simulink model "ElectricalSystem_Test"  (R2019b)
settings: Solver=VariableStepAuto  StartTime=0.0  StopTime=inf  RelTol=1e-3
PostLoadFcn:
  | set_up_test_model
undefined symbols (not defined in the file): AC1CB, AC2CB, AirSupplyIC, APSCB, ATCCabActivation, ATCZeroSpeed, ATOTBDemand, Audio, BLCB, Braking, CECB, CELCB, Class, CMCCB, CRSBCB, CSACB, CSBCB, CSCCB, DeadmanSafetyDevice, DIOCB1, DIOCB2, DLCB, DMICB, Doors, DPLCB, DRCB, EIVIB, ElectricalSystemInput, ElectricalTrainConnection, ElectricalUnitConnection, EmergencyBrakePB, Enabled, ForwardDirection, GrossMass, HasCab, HasMainCompressor, HasMotor, HasPanto, HeadlightSwitch, Height, HLCB, HornPB, ILCB1, ILCB2, IsDM1, IsDM2, IsM1, IsM2, IsT1, IsT2, LeftSideDoorOpen, Length, LoadingMass, MainReservoirPressureSwitch, MasterKeySwitch, MaxVehicles, ModeSelector, NotImmobilise, NotSafetyBrake, NVICB ... (+47)
libraries: TestBenchLib x81
(part 2 of 2)

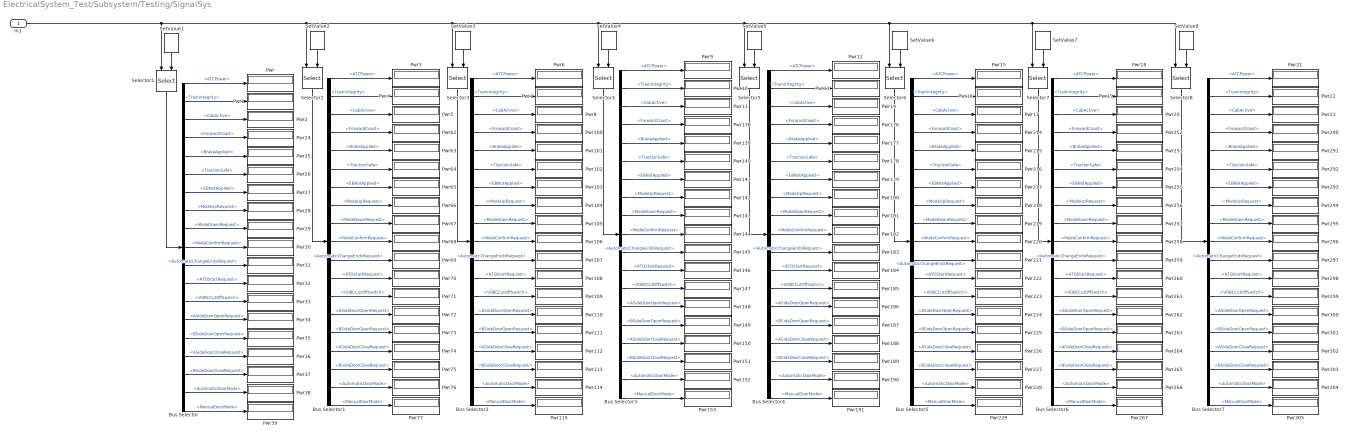
== system ElectricalSystem_Test/Subsystem/Testing/SignalSys ==
  In1 : Inport
  Bus Selector{,1..7} (8 alike) : BusSelector  OutputSignals=SignalSys.ATCPower,SignalSys.TrainIntegrity,SignalSys.CabActive,SignalSys.ForwardCoast,SignalSys.BrakeApplied,SignalSys.TractionSafe,SignalSys.EBNotApplied,SignalSys.ModeUpRequest,SignalSys.ModeDownRequest,SignalSys.ModeConfirmRequest,SignalSys.AutomaticChangeEndsRequest,SignalSys.ATOStartRequest,SignalSys.VOBCCutOffSwitch,SignalSys.ASideDoorOpenRequest,SignalSys.BSideDoorOpenRequest,SignalSys.ASideDoorCloseRequest,SignalSys.BSideDoorCloseRequest,SignalSys.AutomaticDoorMode,SignalSys.ManualDoorMode
  Pwr{,1..39,62..77,100..115,138..153,176..191,214..229,252..267,290..305} (152 alike) : Display
  Selector{1..8} (8 alike) : Selector  InputPortWidth=8  IndexOptions=Index vector (port)  Indices=[1 3]  OutputSizes=1
  SetValue1 : TestBenchLib/SetValue  value=1  init_value=1  WorkspaceVarName=0
      settings: SourceProductName=Sydac Utilities
  SetValue2 : TestBenchLib/SetValue  value=2  init_value=2  WorkspaceVarName=0
      settings: SourceProductName=Sydac Utilities
  SetValue3 : TestBenchLib/SetValue  value=3  init_value=3  WorkspaceVarName=0
      settings: SourceProductName=Sydac Utilities
  SetValue4 : TestBenchLib/SetValue  value=4  init_value=4  WorkspaceVarName=0
      settings: SourceProductName=Sydac Utilities
  SetValue5 : TestBenchLib/SetValue  value=5  init_value=5  WorkspaceVarName=0
      settings: SourceProductName=Sydac Utilities
  SetValue6 : TestBenchLib/SetValue  value=6  init_value=6  WorkspaceVarName=0
      settings: SourceProductName=Sydac Utilities
  SetValue7 : TestBenchLib/SetValue  value=7  init_value=7  WorkspaceVarName=0
      settings: SourceProductName=Sydac Utilities
  SetValue8 : TestBenchLib/SetValue  value=8  init_value=8  WorkspaceVarName=0
      settings: SourceProductName=Sydac Utilities
  wires:
  Selector1/1 -> Bus Selector/1
  SetValue1/1 -> Selector1/2
  Bus Selector/1 -> Pwr/1  "<ATCPower>"
  Bus Selector/2 -> Pwr1/1  "<TrainIntegrity>"
  Bus Selector/3 -> Pwr2/1  "<CabActive>"
  SetValue2/1 -> Selector2/2
  SetValue3/1 -> Selector3/2
  SetValue4/1 -> Selector4/2
  SetValue5/1 -> Selector5/2
  In1/1 -> Selector8/1, Selector7/1, Selector6/1, Selector5/1, Selector4/1, Selector3/1, Selector2/1, Selector1/1
  SetValue6/1 -> Selector6/2
  SetValue7/1 -> Selector7/2
  SetValue8/1 -> Selector8/2
  Bus Selector/4 -> Pwr24/1  "<ForwardCoast>"
  Bus Selector/5 -> Pwr25/1  "<BrakeApplied>"
  Bus Selector/6 -> Pwr26/1  "<TractionSafe>"
  Bus Selector/7 -> Pwr27/1  "<EBNotApplied>"
  Bus Selector/8 -> Pwr28/1  "<ModeUpRequest>"
  Bus Selector/9 -> Pwr29/1  "<ModeDownRequest>"
  Bus Selector/10 -> Pwr30/1  "<ModeConfirmRequest>"
  Bus Selector/11 -> Pwr31/1  "<AutomaticChangeEndsRequest>"
  Bus Selector/12 -> Pwr32/1  "<ATOStartRequest>"
  Bus Selector/13 -> Pwr33/1  "<VOBCCutOffSwitch>"
  Bus Selector/14 -> Pwr34/1  "<ASideDoorOpenRequest>"
  Bus Selector/15 -> Pwr35/1  "<BSideDoorOpenRequest>"
  Bus Selector/16 -> Pwr36/1  "<ASideDoorCloseRequest>"
  Bus Selector/17 -> Pwr37/1  "<BSideDoorCloseRequest>"
  Bus Selector/18 -> Pwr38/1  "<AutomaticDoorMode>"
  Bus Selector/19 -> Pwr39/1  "<ManualDoorMode>"
  Bus Selector1/4 -> Pwr62/1  "<ForwardCoast>"
  Bus Selector1/19 -> Pwr77/1  "<ManualDoorMode>"
  Bus Selector1/17 -> Pwr75/1  "<BSideDoorCloseRequest>"
  Bus Selector1/18 -> Pwr76/1  "<AutomaticDoorMode>"
  Bus Selector1/14 -> Pwr72/1  "<ASideDoorOpenRequest>"
  Bus Selector1/16 -> Pwr74/1  "<ASideDoorCloseRequest>"
  Bus Selector1/15 -> Pwr73/1  "<BSideDoorOpenRequest>"
  Bus Selector1/11 -> Pwr69/1  "<AutomaticChangeEndsRequest>"
  Bus Selector1/13 -> Pwr71/1  "<VOBCCutOffSwitch>"
  Bus Selector1/12 -> Pwr70/1  "<ATOStartRequest>"
  Bus Selector1/9 -> Pwr67/1  "<ModeDownRequest>"
  Bus Selector1/8 -> Pwr66/1  "<ModeUpRequest>"
  Bus Selector1/7 -> Pwr65/1  "<EBNotApplied>"
  Bus Selector1/6 -> Pwr64/1  "<TractionSafe>"
  Bus Selector1/2 -> Pwr4/1  "<TrainIntegrity>"
  Bus Selector1/10 -> Pwr68/1  "<ModeConfirmRequest>"
  Bus Selector1/3 -> Pwr5/1  "<CabActive>"
  Bus Selector1/1 -> Pwr3/1  "<ATCPower>"
  Bus Selector1/5 -> Pwr63/1  "<BrakeApplied>"
  Selector2/1 -> Bus Selector1/1
  Bus Selector2/4 -> Pwr100/1  "<ForwardCoast>"
  Bus Selector2/19 -> Pwr115/1  "<ManualDoorMode>"
  Bus Selector2/17 -> Pwr113/1  "<BSideDoorCloseRequest>"
  Bus Selector2/18 -> Pwr114/1  "<AutomaticDoorMode>"
  Bus Selector2/14 -> Pwr110/1  "<ASideDoorOpenRequest>"
  Bus Selector2/16 -> Pwr112/1  "<ASideDoorCloseRequest>"
  Bus Selector2/15 -> Pwr111/1  "<BSideDoorOpenRequest>"
  Bus Selector2/11 -> Pwr107/1  "<AutomaticChangeEndsRequest>"
  Bus Selector2/13 -> Pwr109/1  "<VOBCCutOffSwitch>"
  Bus Selector2/12 -> Pwr108/1  "<ATOStartRequest>"
  Bus Selector2/9 -> Pwr105/1  "<ModeDownRequest>"
  Bus Selector2/8 -> Pwr104/1  "<ModeUpRequest>"
  Bus Selector2/7 -> Pwr103/1  "<EBNotApplied>"
  Bus Selector2/6 -> Pwr102/1  "<TractionSafe>"
  Bus Selector2/2 -> Pwr7/1  "<TrainIntegrity>"
  Bus Selector2/10 -> Pwr106/1  "<ModeConfirmRequest>"
  Bus Selector2/3 -> Pwr8/1  "<CabActive>"
  Bus Selector2/1 -> Pwr6/1  "<ATCPower>"
  Bus Selector2/5 -> Pwr101/1  "<BrakeApplied>"
  Selector3/1 -> Bus Selector2/1
  Bus Selector3/4 -> Pwr138/1  "<ForwardCoast>"
  Bus Selector3/19 -> Pwr153/1  "<ManualDoorMode>"
  Bus Selector3/17 -> Pwr151/1  "<BSideDoorCloseRequest>"
  Bus Selector3/18 -> Pwr152/1  "<AutomaticDoorMode>"
  Bus Selector3/14 -> Pwr148/1  "<ASideDoorOpenRequest>"
  Bus Selector3/16 -> Pwr150/1  "<ASideDoorCloseRequest>"
  Bus Selector3/15 -> Pwr149/1  "<BSideDoorOpenRequest>"
  Bus Selector3/11 -> Pwr145/1  "<AutomaticChangeEndsRequest>"
  Bus Selector3/13 -> Pwr147/1  "<VOBCCutOffSwitch>"
  Bus Selector3/12 -> Pwr146/1  "<ATOStartRequest>"
  Bus Selector3/9 -> Pwr143/1  "<ModeDownRequest>"
  Bus Selector3/8 -> Pwr142/1  "<ModeUpRequest>"
  Bus Selector3/7 -> Pwr141/1  "<EBNotApplied>"
  Bus Selector3/6 -> Pwr140/1  "<TractionSafe>"
  Bus Selector3/2 -> Pwr10/1  "<TrainIntegrity>"
  Bus Selector3/10 -> Pwr144/1  "<ModeConfirmRequest>"
  Bus Selector3/3 -> Pwr11/1  "<CabActive>"
  Bus Selector3/1 -> Pwr9/1  "<ATCPower>"
  Bus Selector3/5 -> Pwr139/1  "<BrakeApplied>"
  Selector4/1 -> Bus Selector3/1
  Bus Selector4/4 -> Pwr176/1  "<ForwardCoast>"
  Bus Selector4/19 -> Pwr191/1  "<ManualDoorMode>"
  Bus Selector4/17 -> Pwr189/1  "<BSideDoorCloseRequest>"
  Bus Selector4/18 -> Pwr190/1  "<AutomaticDoorMode>"
  Bus Selector4/14 -> Pwr186/1  "<ASideDoorOpenRequest>"
  Bus Selector4/16 -> Pwr188/1  "<ASideDoorCloseRequest>"
  Bus Selector4/15 -> Pwr187/1  "<BSideDoorOpenRequest>"
  Bus Selector4/11 -> Pwr183/1  "<AutomaticChangeEndsRequest>"
  Bus Selector4/13 -> Pwr185/1  "<VOBCCutOffSwitch>"
  Bus Selector4/12 -> Pwr184/1  "<ATOStartRequest>"
  Bus Selector4/9 -> Pwr181/1  "<ModeDownRequest>"
  Bus Selector4/8 -> Pwr180/1  "<ModeUpRequest>"
  Bus Selector4/7 -> Pwr179/1  "<EBNotApplied>"
  Bus Selector4/6 -> Pwr178/1  "<TractionSafe>"
  Bus Selector4/2 -> Pwr13/1  "<TrainIntegrity>"
  Bus Selector4/10 -> Pwr182/1  "<ModeConfirmRequest>"
  Bus Selector4/3 -> Pwr14/1  "<CabActive>"
  Bus Selector4/1 -> Pwr12/1  "<ATCPower>"
  Bus Selector4/5 -> Pwr177/1  "<BrakeApplied>"
  Bus Selector5/4 -> Pwr214/1  "<ForwardCoast>"
  Bus Selector5/19 -> Pwr229/1  "<ManualDoorMode>"
  Bus Selector5/17 -> Pwr227/1  "<BSideDoorCloseRequest>"
  Bus Selector5/18 -> Pwr228/1  "<AutomaticDoorMode>"
  Bus Selector5/14 -> Pwr224/1  "<ASideDoorOpenRequest>"
  Bus Selector5/16 -> Pwr226/1  "<ASideDoorCloseRequest>"
  Bus Selector5/15 -> Pwr225/1  "<BSideDoorOpenRequest>"
  Bus Selector5/11 -> Pwr221/1  "<AutomaticChangeEndsRequest>"
  Bus Selector5/13 -> Pwr223/1  "<VOBCCutOffSwitch>"
  Bus Selector5/12 -> Pwr222/1  "<ATOStartRequest>"
  Bus Selector5/9 -> Pwr219/1  "<ModeDownRequest>"
  Bus Selector5/8 -> Pwr218/1  "<ModeUpRequest>"
  Bus Selector5/7 -> Pwr217/1  "<EBNotApplied>"
  Bus Selector5/6 -> Pwr216/1  "<TractionSafe>"
  Bus Selector5/2 -> Pwr16/1  "<TrainIntegrity>"
  Bus Selector5/10 -> Pwr220/1  "<ModeConfirmRequest>"
  Bus Selector5/3 -> Pwr17/1  "<CabActive>"
  Bus Selector5/1 -> Pwr15/1  "<ATCPower>"
  Bus Selector5/5 -> Pwr215/1  "<BrakeApplied>"
  Selector6/1 -> Bus Selector5/1
  Bus Selector6/4 -> Pwr252/1  "<ForwardCoast>"
  Bus Selector6/19 -> Pwr267/1  "<ManualDoorMode>"
  Bus Selector6/17 -> Pwr265/1  "<BSideDoorCloseRequest>"
  Bus Selector6/18 -> Pwr266/1  "<AutomaticDoorMode>"
  Bus Selector6/14 -> Pwr262/1  "<ASideDoorOpenRequest>"
  Bus Selector6/16 -> Pwr264/1  "<ASideDoorCloseRequest>"
  Bus Selector6/15 -> Pwr263/1  "<BSideDoorOpenRequest>"
  Bus Selector6/11 -> Pwr259/1  "<AutomaticChangeEndsRequest>"
  Bus Selector6/13 -> Pwr261/1  "<VOBCCutOffSwitch>"
  Bus Selector6/12 -> Pwr260/1  "<ATOStartRequest>"
  Bus Selector6/9 -> Pwr257/1  "<ModeDownRequest>"
  Bus Selector6/8 -> Pwr256/1  "<ModeUpRequest>"
  Bus Selector6/7 -> Pwr255/1  "<EBNotApplied>"
  Bus Selector6/6 -> Pwr254/1  "<TractionSafe>"
  Bus Selector6/2 -> Pwr19/1  "<TrainIntegrity>"
  Bus Selector6/10 -> Pwr258/1  "<ModeConfirmRequest>"
  Bus Selector6/3 -> Pwr20/1  "<CabActive>"
  Bus Selector6/1 -> Pwr18/1  "<ATCPower>"
  Bus Selector6/5 -> Pwr253/1  "<BrakeApplied>"
  Selector7/1 -> Bus Selector6/1
  Bus Selector7/4 -> Pwr290/1  "<ForwardCoast>"
  Bus Selector7/19 -> Pwr305/1  "<ManualDoorMode>"
  Bus Selector7/17 -> Pwr303/1  "<BSideDoorCloseRequest>"
  Bus Selector7/18 -> Pwr304/1  "<AutomaticDoorMode>"
  Bus Selector7/14 -> Pwr300/1  "<ASideDoorOpenRequest>"
  Bus Selector7/16 -> Pwr302/1  "<ASideDoorCloseRequest>"
  Bus Selector7/15 -> Pwr301/1  "<BSideDoorOpenRequest>"
  Bus Selector7/11 -> Pwr297/1  "<AutomaticChangeEndsRequest>"
  Bus Selector7/13 -> Pwr299/1  "<VOBCCutOffSwitch>"
  Bus Selector7/12 -> Pwr298/1  "<ATOStartRequest>"
  Bus Selector7/9 -> Pwr295/1  "<ModeDownRequest>"
  Bus Selector7/8 -> Pwr294/1  "<ModeUpRequest>"
  Bus Selector7/7 -> Pwr293/1  "<EBNotApplied>"
  Bus Selector7/6 -> Pwr292/1  "<TractionSafe>"
  Bus Selector7/2 -> Pwr22/1  "<TrainIntegrity>"
  Bus Selector7/10 -> Pwr296/1  "<ModeConfirmRequest>"
  Bus Selector7/3 -> Pwr23/1  "<CabActive>"
  Bus Selector7/1 -> Pwr21/1  "<ATCPower>"
  Bus Selector7/5 -> Pwr291/1  "<BrakeApplied>"
  Selector8/1 -> Bus Selector7/1
  Selector5/1 -> Bus Selector4/1

== system ElectricalSystem_Test/Subsystem/Testing/Subsystem ==
  In1 : Inport
  Bus Creator : BusCreator  Inputs=OutputControlStates,Traction,Braking,TCMS,Pneumatics,SignalSys,Doors,Audio
  For Each Subsystem : Subsystem  TreatAsAtomicUnit=on
  Out1 : Outport
  wires:
  In1/1 -> For Each Subsystem/1(In1)
  For Each Subsystem/1(Out1) -> Bus Creator/1  "OutputControlStates"
  For Each Subsystem/2(Out2) -> Bus Creator/2  "Traction"
  For Each Subsystem/3(Out3) -> Bus Creator/3  "Braking"
  For Each Subsystem/4(Out5) -> Bus Creator/4  "TCMS"
  For Each Subsystem/5(Out6) -> Bus Creator/5  "Pneumatics"
  For Each Subsystem/6(Out7) -> Bus Creator/6  "SignalSys"
  For Each Subsystem/7(Out8) -> Bus Creator/7  "Doors"
  Bus Creator/1 -> Out1/1
  For Each Subsystem/8(Out4) -> Bus Creator/8  "Audio"

== system ElectricalSystem_Test/Subsystem/Testing/Subsystem1 ==
  In1 : Inport  Partition=on  PartitionDimension=1  PartitionWidth=1  PartitionOffset=0
  In2 : Inport  Port=2  Partition=on  PartitionDimension=1  PartitionWidth=1  PartitionOffset=0
  Bus Assignment4 : BusAssignment  AssignedSignals=ElectricalUnitConnection,ElectricalTrainConnection
  Constant5 : Constant  Value=0  OutDataTypeStr=Bus: BD_ElectricalSystem_In_Vehicle_Coupling
  For Each : ForEach  DisableCoverage=on
  Out1 : Outport  ConcatenationDimension=1
  wires:
  Constant5/1 -> Bus Assignment4/1
  In1/1 -> Bus Assignment4/2
  Bus Assignment4/1 -> Out1/1
  In2/1 -> Bus Assignment4/3

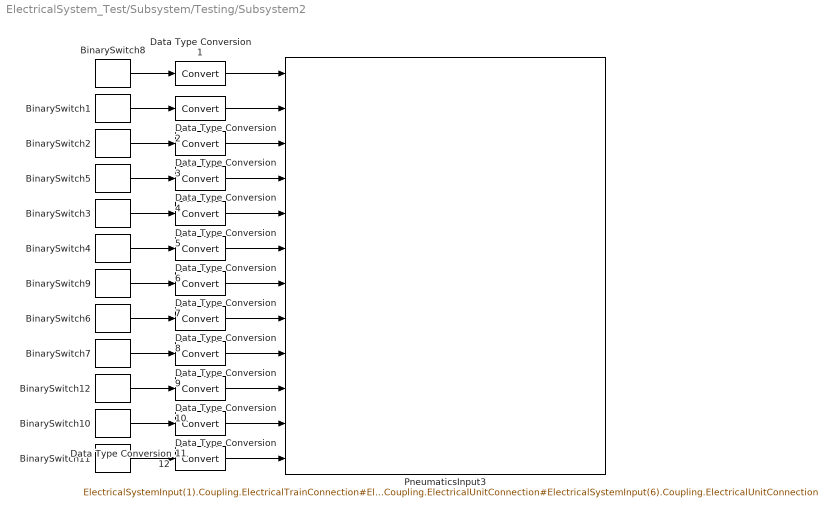
== system ElectricalSystem_Test/Subsystem/Testing/Subsystem2 ==
  BinarySwitch{1..7,10..11} (9 alike) : TestBenchLib/BinarySwitch  value=1  init_value=1  block_colour=[0 1 0]  WorkspaceVarName=0
      settings: SourceProductName=Sydac Utilities
  BinarySwitch12 : TestBenchLib/BinarySwitch  value=0  init_value=0  block_colour=[0 1 0]  WorkspaceVarName=0
      settings: SourceProductName=Sydac Utilities
  BinarySwitch8 : TestBenchLib/BinarySwitch  value=0  init_value=0  block_colour=[0 1 0]  WorkspaceVarName=0
      settings: SourceProductName=Sydac Utilities
  BinarySwitch9 : TestBenchLib/BinarySwitch  value=0  init_value=0  block_colour=[0 1 0]  WorkspaceVarName=0
      settings: SourceProductName=Sydac Utilities
  Data Type Conversion{1..12} (12 alike) : DataTypeConversion
  PneumaticsInput3 : DataStoreWrite  DataStoreName=ElectricalSystemInput  DataStoreElements=ElectricalSystemInput(1).Coupling.ElectricalTrainConnection#ElectricalSystemInput(2).Coupling.ElectricalTrainConnection#ElectricalSystemInput(3).Coupling.ElectricalTrainConnection#ElectricalSystemInput(4).Coupling.ElectricalTrainConnection#ElectricalSystemInput(5).Coupling.ElectricalTrainConnection#ElectricalSystemInput(6).Coupling.ElectricalTrainConnection#ElectricalSystemInput(1).Coupling.ElectricalUnitConnection#ElectricalSystemInput(2).Coupling.ElectricalUnitConnection#ElectricalSystemInput(3).Coupling.ElectricalUnitConnection#ElectricalSystemInput(4).Coupling.ElectricalUnitConnection#ElectricalSystemInput(5).Coupling.ElectricalUnitConnection#ElectricalSystemInput(6).Coupling.ElectricalUnitConnection
  wires:
  Data Type Conversion1/1 -> PneumaticsInput3/1
  BinarySwitch8/1 -> Data Type Conversion1/1
  BinarySwitch1/1 -> Data Type Conversion2/1
  Data Type Conversion2/1 -> PneumaticsInput3/2
  BinarySwitch2/1 -> Data Type Conversion3/1
  Data Type Conversion3/1 -> PneumaticsInput3/3
  Data Type Conversion6/1 -> PneumaticsInput3/6
  BinarySwitch4/1 -> Data Type Conversion6/1
  Data Type Conversion5/1 -> PneumaticsInput3/5
  BinarySwitch3/1 -> Data Type Conversion5/1
  BinarySwitch5/1 -> Data Type Conversion4/1
  Data Type Conversion4/1 -> PneumaticsInput3/4
  BinarySwitch9/1 -> Data Type Conversion7/1
  BinarySwitch6/1 -> Data Type Conversion8/1
  BinarySwitch7/1 -> Data Type Conversion9/1
  Data Type Conversion9/1 -> PneumaticsInput3/9
  Data Type Conversion8/1 -> PneumaticsInput3/8
  Data Type Conversion7/1 -> PneumaticsInput3/7
  Data Type Conversion11/1 -> PneumaticsInput3/11
  Data Type Conversion12/1 -> PneumaticsInput3/12
  BinarySwitch11/1 -> Data Type Conversion12/1
  BinarySwitch10/1 -> Data Type Conversion11/1
  Data Type Conversion10/1 -> PneumaticsInput3/10
  BinarySwitch12/1 -> Data Type Conversion10/1

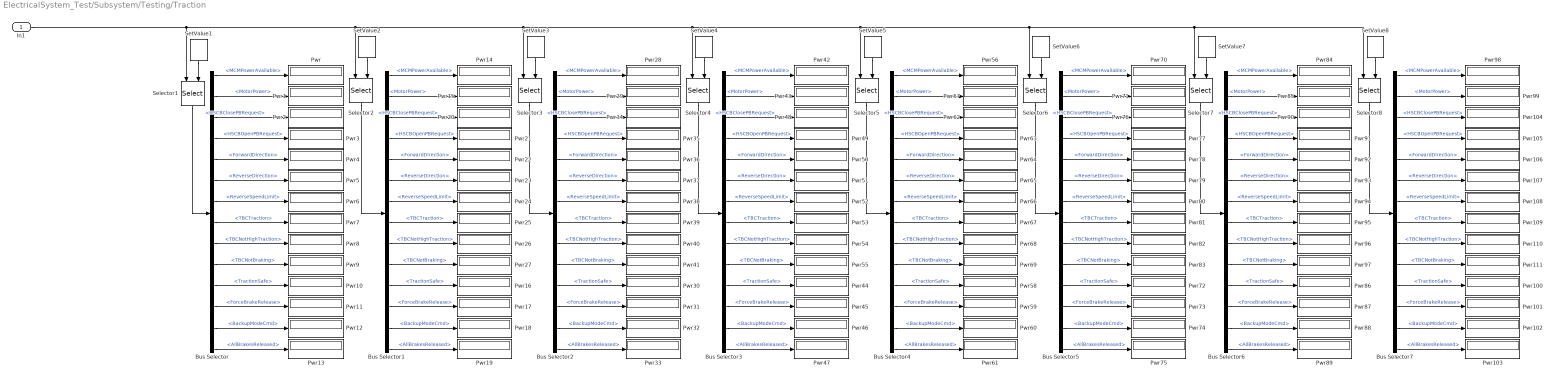
== system ElectricalSystem_Test/Subsystem/Testing/Traction ==
  In1 : Inport
  Bus Selector{,1..7} (8 alike) : BusSelector  OutputSignals=Traction.MCMPowerAvailable,Traction.MotorPower,Traction.HSCBClosePBRequest,Traction.HSCBOpenPBRequest,Traction.ForwardDirection,Traction.ReverseDirection,Traction.ReverseSpeedLimit,Traction.TBCTraction,Traction.TBCNotHighTraction,Traction.TBCNotBraking,Traction.TractionSafe,Traction.ForceBrakeRelease,Traction.BackupModeCmd,Traction.AllBrakesReleased
  Pwr{,1..111} (112 alike) : Display
  Selector{1..8} (8 alike) : Selector  InputPortWidth=8  IndexOptions=Index vector (port)  Indices=[1 3]  OutputSizes=1
  SetValue1 : TestBenchLib/SetValue  value=1  init_value=1  WorkspaceVarName=0
      settings: SourceProductName=Sydac Utilities
  SetValue2 : TestBenchLib/SetValue  value=2  init_value=2  WorkspaceVarName=0
      settings: SourceProductName=Sydac Utilities
  SetValue3 : TestBenchLib/SetValue  value=3  init_value=3  WorkspaceVarName=0
      settings: SourceProductName=Sydac Utilities
  SetValue4 : TestBenchLib/SetValue  value=4  init_value=4  WorkspaceVarName=0
      settings: SourceProductName=Sydac Utilities
  SetValue5 : TestBenchLib/SetValue  value=5  init_value=5  WorkspaceVarName=0
      settings: SourceProductName=Sydac Utilities
  SetValue6 : TestBenchLib/SetValue  value=6  init_value=6  WorkspaceVarName=0
      settings: SourceProductName=Sydac Utilities
  SetValue7 : TestBenchLib/SetValue  value=7  init_value=7  WorkspaceVarName=0
      settings: SourceProductName=Sydac Utilities
  SetValue8 : TestBenchLib/SetValue  value=8  init_value=8  WorkspaceVarName=0
      settings: SourceProductName=Sydac Utilities
  wires:
  Selector1/1 -> Bus Selector/1
  SetValue1/1 -> Selector1/2
  Bus Selector/1 -> Pwr/1  "<MCMPowerAvailable>"
  Bus Selector/2 -> Pwr1/1  "<MotorPower>"
  Bus Selector/3 -> Pwr2/1  "<HSCBClosePBRequest>"
  Bus Selector/4 -> Pwr3/1  "<HSCBOpenPBRequest>"
  Bus Selector/5 -> Pwr4/1  "<ForwardDirection>"
  Bus Selector/6 -> Pwr5/1  "<ReverseDirection>"
  Bus Selector/7 -> Pwr6/1  "<ReverseSpeedLimit>"
  Bus Selector/8 -> Pwr7/1  "<TBCTraction>"
  Bus Selector/9 -> Pwr8/1  "<TBCNotHighTraction>"
  Bus Selector/10 -> Pwr9/1  "<TBCNotBraking>"
  Bus Selector/11 -> Pwr10/1  "<TractionSafe>"
  Bus Selector/12 -> Pwr11/1  "<ForceBrakeRelease>"
  Bus Selector/13 -> Pwr12/1  "<BackupModeCmd>"
  Bus Selector/14 -> Pwr13/1  "<AllBrakesReleased>"
  Bus Selector1/14 -> Pwr19/1  "<AllBrakesReleased>"
  Bus Selector1/13 -> Pwr18/1  "<BackupModeCmd>"
  Bus Selector1/12 -> Pwr17/1  "<ForceBrakeRelease>"
  Bus Selector1/11 -> Pwr16/1  "<TractionSafe>"
  Bus Selector1/10 -> Pwr27/1  "<TBCNotBraking>"
  Bus Selector1/9 -> Pwr26/1  "<TBCNotHighTraction>"
  Bus Selector1/8 -> Pwr25/1  "<TBCTraction>"
  Bus Selector1/7 -> Pwr24/1  "<ReverseSpeedLimit>"
  Bus Selector1/6 -> Pwr23/1  "<ReverseDirection>"
  Bus Selector1/5 -> Pwr22/1  "<ForwardDirection>"
  Bus Selector1/4 -> Pwr21/1  "<HSCBOpenPBRequest>"
  Bus Selector1/3 -> Pwr20/1  "<HSCBClosePBRequest>"
  Bus Selector1/2 -> Pwr15/1  "<MotorPower>"
  Bus Selector1/1 -> Pwr14/1  "<MCMPowerAvailable>"
  Selector2/1 -> Bus Selector1/1
  SetValue2/1 -> Selector2/2
  SetValue3/1 -> Selector3/2
  Selector3/1 -> Bus Selector2/1
  Bus Selector2/1 -> Pwr28/1  "<MCMPowerAvailable>"
  Bus Selector2/2 -> Pwr29/1  "<MotorPower>"
  Bus Selector2/3 -> Pwr34/1  "<HSCBClosePBRequest>"
  Bus Selector2/4 -> Pwr35/1  "<HSCBOpenPBRequest>"
  Bus Selector2/5 -> Pwr36/1  "<ForwardDirection>"
  Bus Selector2/6 -> Pwr37/1  "<ReverseDirection>"
  Bus Selector2/7 -> Pwr38/1  "<ReverseSpeedLimit>"
  Bus Selector2/8 -> Pwr39/1  "<TBCTraction>"
  Bus Selector2/9 -> Pwr40/1  "<TBCNotHighTraction>"
  Bus Selector2/10 -> Pwr41/1  "<TBCNotBraking>"
  Bus Selector2/11 -> Pwr30/1  "<TractionSafe>"
  Bus Selector2/12 -> Pwr31/1  "<ForceBrakeRelease>"
  Bus Selector2/13 -> Pwr32/1  "<BackupModeCmd>"
  Bus Selector2/14 -> Pwr33/1  "<AllBrakesReleased>"
  Bus Selector3/14 -> Pwr47/1  "<AllBrakesReleased>"
  Bus Selector3/13 -> Pwr46/1  "<BackupModeCmd>"
  Bus Selector3/12 -> Pwr45/1  "<ForceBrakeRelease>"
  Bus Selector3/11 -> Pwr44/1  "<TractionSafe>"
  Bus Selector3/10 -> Pwr55/1  "<TBCNotBraking>"
  Bus Selector3/9 -> Pwr54/1  "<TBCNotHighTraction>"
  Bus Selector3/8 -> Pwr53/1  "<TBCTraction>"
  Bus Selector3/7 -> Pwr52/1  "<ReverseSpeedLimit>"
  Bus Selector3/6 -> Pwr51/1  "<ReverseDirection>"
  Bus Selector3/5 -> Pwr50/1  "<ForwardDirection>"
  Bus Selector3/4 -> Pwr49/1  "<HSCBOpenPBRequest>"
  Bus Selector3/3 -> Pwr48/1  "<HSCBClosePBRequest>"
  Bus Selector3/2 -> Pwr43/1  "<MotorPower>"
  Bus Selector3/1 -> Pwr42/1  "<MCMPowerAvailable>"
  Selector4/1 -> Bus Selector3/1
  SetValue4/1 -> Selector4/2
  SetValue5/1 -> Selector5/2
  Selector5/1 -> Bus Selector4/1
  Bus Selector4/1 -> Pwr56/1  "<MCMPowerAvailable>"
  Bus Selector4/2 -> Pwr57/1  "<MotorPower>"
  Bus Selector4/3 -> Pwr62/1  "<HSCBClosePBRequest>"
  Bus Selector4/4 -> Pwr63/1  "<HSCBOpenPBRequest>"
  Bus Selector4/5 -> Pwr64/1  "<ForwardDirection>"
  Bus Selector4/6 -> Pwr65/1  "<ReverseDirection>"
  Bus Selector4/7 -> Pwr66/1  "<ReverseSpeedLimit>"
  Bus Selector4/8 -> Pwr67/1  "<TBCTraction>"
  Bus Selector4/9 -> Pwr68/1  "<TBCNotHighTraction>"
  Bus Selector4/10 -> Pwr69/1  "<TBCNotBraking>"
  Bus Selector4/11 -> Pwr58/1  "<TractionSafe>"
  Bus Selector4/12 -> Pwr59/1  "<ForceBrakeRelease>"
  Bus Selector4/13 -> Pwr60/1  "<BackupModeCmd>"
  Bus Selector4/14 -> Pwr61/1  "<AllBrakesReleased>"
  In1/1 -> Selector8/1, Selector7/1, Selector6/1, Selector5/1, Selector4/1, Selector3/1, Selector2/1, Selector1/1
  Bus Selector5/14 -> Pwr75/1  "<AllBrakesReleased>"
  Bus Selector5/13 -> Pwr74/1  "<BackupModeCmd>"
  Bus Selector5/12 -> Pwr73/1  "<ForceBrakeRelease>"
  Bus Selector5/11 -> Pwr72/1  "<TractionSafe>"
  Bus Selector5/10 -> Pwr83/1  "<TBCNotBraking>"
  Bus Selector5/9 -> Pwr82/1  "<TBCNotHighTraction>"
  Bus Selector5/8 -> Pwr81/1  "<TBCTraction>"
  Bus Selector5/7 -> Pwr80/1  "<ReverseSpeedLimit>"
  Bus Selector5/6 -> Pwr79/1  "<ReverseDirection>"
  Bus Selector5/5 -> Pwr78/1  "<ForwardDirection>"
  Bus Selector5/4 -> Pwr77/1  "<HSCBOpenPBRequest>"
  Bus Selector5/3 -> Pwr76/1  "<HSCBClosePBRequest>"
  Bus Selector5/2 -> Pwr71/1  "<MotorPower>"
  Bus Selector5/1 -> Pwr70/1  "<MCMPowerAvailable>"
  Selector6/1 -> Bus Selector5/1
  SetValue6/1 -> Selector6/2
  SetValue7/1 -> Selector7/2
  Selector7/1 -> Bus Selector6/1
  Bus Selector6/1 -> Pwr84/1  "<MCMPowerAvailable>"
  Bus Selector6/2 -> Pwr85/1  "<MotorPower>"
  Bus Selector6/3 -> Pwr90/1  "<HSCBClosePBRequest>"
  Bus Selector6/4 -> Pwr91/1  "<HSCBOpenPBRequest>"
  Bus Selector6/5 -> Pwr92/1  "<ForwardDirection>"
  Bus Selector6/6 -> Pwr93/1  "<ReverseDirection>"
  Bus Selector6/7 -> Pwr94/1  "<ReverseSpeedLimit>"
  Bus Selector6/8 -> Pwr95/1  "<TBCTraction>"
  Bus Selector6/9 -> Pwr96/1  "<TBCNotHighTraction>"
  Bus Selector6/10 -> Pwr97/1  "<TBCNotBraking>"
  Bus Selector6/11 -> Pwr86/1  "<TractionSafe>"
  Bus Selector6/12 -> Pwr87/1  "<ForceBrakeRelease>"
  Bus Selector6/13 -> Pwr88/1  "<BackupModeCmd>"
  Bus Selector6/14 -> Pwr89/1  "<AllBrakesReleased>"
  Bus Selector7/14 -> Pwr103/1  "<AllBrakesReleased>"
  Bus Selector7/13 -> Pwr102/1  "<BackupModeCmd>"
  Bus Selector7/12 -> Pwr101/1  "<ForceBrakeRelease>"
  Bus Selector7/11 -> Pwr100/1  "<TractionSafe>"
  Bus Selector7/10 -> Pwr111/1  "<TBCNotBraking>"
  Bus Selector7/9 -> Pwr110/1  "<TBCNotHighTraction>"
  Bus Selector7/8 -> Pwr109/1  "<TBCTraction>"
  Bus Selector7/7 -> Pwr108/1  "<ReverseSpeedLimit>"
  Bus Selector7/6 -> Pwr107/1  "<ReverseDirection>"
  Bus Selector7/5 -> Pwr106/1  "<ForwardDirection>"
  Bus Selector7/4 -> Pwr105/1  "<HSCBOpenPBRequest>"
  Bus Selector7/3 -> Pwr104/1  "<HSCBClosePBRequest>"
  Bus Selector7/2 -> Pwr99/1  "<MotorPower>"
  Bus Selector7/1 -> Pwr98/1  "<MCMPowerAvailable>"
  Selector8/1 -> Bus Selector7/1
  SetValue8/1 -> Selector8/2

== system ElectricalSystem_Test/Subsystem/Testing/BD_ElectricalSystem_Out_Vehicle_Audio/ExtractData ==
  In1 : Inport  Partition=on  PartitionDimension=1  PartitionWidth=1  PartitionOffset=0
  Bus Selector : BusSelector  OutputSignals=Horn,VigilanceBuzzer,PantographGroundFaultNoise,PantographGroundFaultNoiseVolume
  For Each : ForEach  DisableCoverage=on
  Out1 : Outport  ConcatenationDimension=1
  Out2 : Outport  Port=2  ConcatenationDimension=1
  Out3 : Outport  Port=3  ConcatenationDimension=1
  Out4 : Outport  Port=4  ConcatenationDimension=1
  wires:
  Bus Selector/3 -> Out3/1  "<PantographGroundFaultNoise>"
  Bus Selector/2 -> Out2/1  "<VigilanceBuzzer>"
  Bus Selector/1 -> Out1/1  "<Horn>"
  In1/1 -> Bus Selector/1
  Bus Selector/4 -> Out4/1  "<PantographGroundFaultNoiseVolume>"

== system ElectricalSystem_Test/Subsystem/Testing/BD_ElectricalSystem_Out_Vehicle_Braking/ExtractData ==
  In1 : Inport  Partition=on  PartitionDimension=1  PartitionWidth=1  PartitionOffset=0
  Bus Selector : BusSelector  OutputSignals=BCUPower,TBCTraction,TBCNotBraking,TBCNotHighBrake,ForceBrakeReleaseCmd,BackupModeCmd,NoEB,BrakeControlNotIsolated
  For Each : ForEach  DisableCoverage=on
  Power : Outport  ConcatenationDimension=1
  Traction : Outport  Port=2  ConcatenationDimension=1
  Braking : Outport  Port=3  ConcatenationDimension=1
  Not High Braking : Outport  Port=4  ConcatenationDimension=1
  Force Brake Release Cmd : Outport  Port=5  ConcatenationDimension=1
  Backup Mode : Outport  Port=6  ConcatenationDimension=1
  NoEB : Outport  Port=7  ConcatenationDimension=1
  NoEB1 : Outport  Port=8  ConcatenationDimension=1
  wires:
  In1/1 -> Bus Selector/1
  Bus Selector/1 -> Power/1  "<BCUPower>"
  Bus Selector/2 -> Traction/1  "<TBCTraction>"
  Bus Selector/3 -> Braking/1  "<TBCNotBraking>"
  Bus Selector/4 -> Not High Braking/1  "<TBCNotHighBrake>"
  Bus Selector/5 -> Force Brake Release Cmd/1  "<ForceBrakeReleaseCmd>"
  Bus Selector/6 -> Backup Mode/1  "<BackupModeCmd>"
  Bus Selector/7 -> NoEB/1  "<NoEB>"
  Bus Selector/8 -> NoEB1/1  "<BrakeControlNotIsolated>"

== system ElectricalSystem_Test/Subsystem/Testing/BD_ElectricalSystem_Out_Vehicle_Doors/ExtractData ==
  In1 : Inport  Partition=on  PartitionDimension=1  PartitionWidth=1  PartitionOffset=0
  Bus Selector : BusSelector  OutputSignals=ASideDoorOpenRequest,BSideDoorOpenRequest,ASideDoorCloseRequest,BSideDoorCloseRequest,ASideDoorEnable,BSideDoorEnable,ZeroSpeed,DCUPower
  For Each : ForEach  DisableCoverage=on
  Out1 : Outport  ConcatenationDimension=1
  Out2 : Outport  Port=2  ConcatenationDimension=1
  Out3 : Outport  Port=3  ConcatenationDimension=1
  Out4 : Outport  Port=4  ConcatenationDimension=1
  Out5 : Outport  Port=5  ConcatenationDimension=1
  Out6 : Outport  Port=6  ConcatenationDimension=1
  Out7 : Outport  Port=7  ConcatenationDimension=1
  Out8 : Outport  Port=8  ConcatenationDimension=1
  wires:
  In1/1 -> Bus Selector/1
  Bus Selector/1 -> Out1/1  "<ASideDoorOpenRequest>"
  Bus Selector/2 -> Out2/1  "<BSideDoorOpenRequest>"
  Bus Selector/3 -> Out3/1  "<ASideDoorCloseRequest>"
  Bus Selector/4 -> Out4/1  "<BSideDoorCloseRequest>"
  Bus Selector/5 -> Out5/1  "<ASideDoorEnable>"
  Bus Selector/6 -> Out6/1  "<BSideDoorEnable>"
  Bus Selector/7 -> Out7/1  "<ZeroSpeed>"
  Bus Selector/8 -> Out8/1  "<DCUPower>"

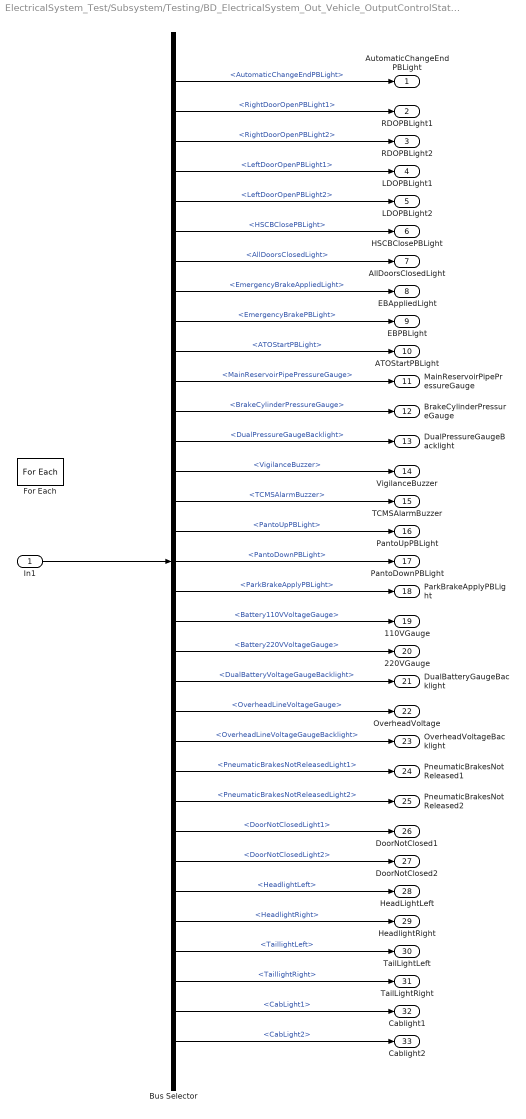
== system ElectricalSystem_Test/Subsystem/Testing/BD_ElectricalSystem_Out_Vehicle_OutputControlStates/ExtractData ==
  In1 : Inport  Partition=on  PartitionDimension=1  PartitionWidth=1  PartitionOffset=0
  Bus Selector : BusSelector  OutputSignals=AutomaticChangeEndPBLight,RightDoorOpenPBLight1,RightDoorOpenPBLight2,LeftDoorOpenPBLight1,LeftDoorOpenPBLight2,HSCBClosePBLight,AllDoorsClosedLight,EmergencyBrakeAppliedLight,EmergencyBrakePBLight,ATOStartPBLight,MainReservoirPipePressureGauge,BrakeCylinderPressureGauge,DualPressureGaugeBacklight,VigilanceBuzzer,TCMSAlarmBuzzer,PantoUpPBLight,PantoDownPBLight,ParkBrakeApplyPBLight,Battery110VVoltageGauge,Battery220VVoltageGauge,DualBatteryVoltageGaugeBacklight,OverheadLineVoltageGauge,OverheadLineVoltageGaugeBacklight,PneumaticBrakesNotReleasedLight1,PneumaticBrakesNotReleasedLight2,DoorNotClosedLight1,DoorNotClosedLight2,HeadlightLeft,HeadlightRight,TaillightLeft,TaillightRight,CabLight1,CabLight2
  For Each : ForEach  DisableCoverage=on
  AutomaticChangeEndPBLight : Outport  ConcatenationDimension=1
  RDOPBLight1 : Outport  Port=2  ConcatenationDimension=1
  RDOPBLight2 : Outport  Port=3  ConcatenationDimension=1
  LDOPBLight1 : Outport  Port=4  ConcatenationDimension=1
  LDOPBLight2 : Outport  Port=5  ConcatenationDimension=1
  HSCBClosePBLight : Outport  Port=6  ConcatenationDimension=1
  AllDoorsClosedLight : Outport  Port=7  ConcatenationDimension=1
  EBAppliedLight : Outport  Port=8  ConcatenationDimension=1
  EBPBLight : Outport  Port=9  ConcatenationDimension=1
  ATOStartPBLight : Outport  Port=10  ConcatenationDimension=1
  MainReservoirPipePressureGauge : Outport  Port=11  ConcatenationDimension=1
  BrakeCylinderPressureGauge : Outport  Port=12  ConcatenationDimension=1
  DualPressureGaugeBacklight : Outport  Port=13  ConcatenationDimension=1
  VigilanceBuzzer : Outport  Port=14  ConcatenationDimension=1
  TCMSAlarmBuzzer : Outport  Port=15  ConcatenationDimension=1
  PantoUpPBLight : Outport  Port=16  ConcatenationDimension=1
  PantoDownPBLight : Outport  Port=17  ConcatenationDimension=1
  ParkBrakeApplyPBLight : Outport  Port=18  ConcatenationDimension=1
  110VGauge : Outport  Port=19  ConcatenationDimension=1
  220VGauge : Outport  Port=20  ConcatenationDimension=1
  DualBatteryGaugeBacklight : Outport  Port=21  ConcatenationDimension=1
  OverheadVoltage : Outport  Port=22  ConcatenationDimension=1
  OverheadVoltageBacklight : Outport  Port=23  ConcatenationDimension=1
  PneumaticBrakesNotReleased1 : Outport  Port=24  ConcatenationDimension=1
  PneumaticBrakesNotReleased2 : Outport  Port=25  ConcatenationDimension=1
  DoorNotClosed1 : Outport  Port=26  ConcatenationDimension=1
  DoorNotClosed2 : Outport  Port=27  ConcatenationDimension=1
  HeadLightLeft : Outport  Port=28  ConcatenationDimension=1
  HeadlightRight : Outport  Port=29  ConcatenationDimension=1
  TailLightLeft : Outport  Port=30  ConcatenationDimension=1
  TailLightRight : Outport  Port=31  ConcatenationDimension=1
  Cablight1 : Outport  Port=32  ConcatenationDimension=1
  Cablight2 : Outport  Port=33  ConcatenationDimension=1
  wires:
  Bus Selector/16 -> PantoUpPBLight/1  "<PantoUpPBLight>"
  Bus Selector/15 -> TCMSAlarmBuzzer/1  "<TCMSAlarmBuzzer>"
  Bus Selector/14 -> VigilanceBuzzer/1  "<VigilanceBuzzer>"
  In1/1 -> Bus Selector/1
  Bus Selector/1 -> AutomaticChangeEndPBLight/1  "<AutomaticChangeEndPBLight>"
  Bus Selector/6 -> HSCBClosePBLight/1  "<HSCBClosePBLight>"
  Bus Selector/7 -> AllDoorsClosedLight/1  "<AllDoorsClosedLight>"
  Bus Selector/8 -> EBAppliedLight/1  "<EmergencyBrakeAppliedLight>"
  Bus Selector/9 -> EBPBLight/1  "<EmergencyBrakePBLight>"
  Bus Selector/10 -> ATOStartPBLight/1  "<ATOStartPBLight>"
  Bus Selector/11 -> MainReservoirPipePressureGauge/1  "<MainReservoirPipePressureGauge>"
  Bus Selector/12 -> BrakeCylinderPressureGauge/1  "<BrakeCylinderPressureGauge>"
  Bus Selector/13 -> DualPressureGaugeBacklight/1  "<DualPressureGaugeBacklight>"
  Bus Selector/17 -> PantoDownPBLight/1  "<PantoDownPBLight>"
  Bus Selector/18 -> ParkBrakeApplyPBLight/1  "<ParkBrakeApplyPBLight>"
  Bus Selector/19 -> 110VGauge/1  "<Battery110VVoltageGauge>"
  Bus Selector/20 -> 220VGauge/1  "<Battery220VVoltageGauge>"
  Bus Selector/21 -> DualBatteryGaugeBacklight/1  "<DualBatteryVoltageGaugeBacklight>"
  Bus Selector/22 -> OverheadVoltage/1  "<OverheadLineVoltageGauge>"
  Bus Selector/23 -> OverheadVoltageBacklight/1  "<OverheadLineVoltageGaugeBacklight>"
  Bus Selector/24 -> PneumaticBrakesNotReleased1/1  "<PneumaticBrakesNotReleasedLight1>"
  Bus Selector/25 -> PneumaticBrakesNotReleased2/1  "<PneumaticBrakesNotReleasedLight2>"
  Bus Selector/26 -> DoorNotClosed1/1  "<DoorNotClosedLight1>"
  Bus Selector/27 -> DoorNotClosed2/1  "<DoorNotClosedLight2>"
  Bus Selector/28 -> HeadLightLeft/1  "<HeadlightLeft>"
  Bus Selector/31 -> TailLightRight/1  "<TaillightRight>"
  Bus Selector/30 -> TailLightLeft/1  "<TaillightLeft>"
  Bus Selector/29 -> HeadlightRight/1  "<HeadlightRight>"
  Bus Selector/32 -> Cablight1/1  "<CabLight1>"
  Bus Selector/33 -> Cablight2/1  "<CabLight2>"
  Bus Selector/2 -> RDOPBLight1/1  "<RightDoorOpenPBLight1>"
  Bus Selector/3 -> RDOPBLight2/1  "<RightDoorOpenPBLight2>"
  Bus Selector/4 -> LDOPBLight1/1  "<LeftDoorOpenPBLight1>"
  Bus Selector/5 -> LDOPBLight2/1  "<LeftDoorOpenPBLight2>"

== system ElectricalSystem_Test/Subsystem/Testing/BD_ElectricalSystem_Out_Vehicle_Pneumatics/ExtractData ==
  In1 : Inport  Partition=on  PartitionDimension=1  PartitionWidth=1  PartitionOffset=0
  Bus Selector : BusSelector  OutputSignals=PantoUpCmd,PantoDownCmd,ParkBrakeApplyCmd,ParkBrakeReleaseCmd,AirCompressorMotorPower
  For Each : ForEach  DisableCoverage=on
  Out1 : Outport  ConcatenationDimension=1
  Out2 : Outport  Port=2  ConcatenationDimension=1
  Out4 : Outport  Port=3  ConcatenationDimension=1
  Out5 : Outport  Port=4  ConcatenationDimension=1
  Out3 : Outport  Port=5  ConcatenationDimension=1
  wires:
  In1/1 -> Bus Selector/1
  Bus Selector/1 -> Out1/1  "<PantoUpCmd>"
  Bus Selector/2 -> Out2/1  "<PantoDownCmd>"
  Bus Selector/5 -> Out3/1  "<AirCompressorMotorPower>"
  Bus Selector/4 -> Out5/1  "<ParkBrakeReleaseCmd>"
  Bus Selector/3 -> Out4/1  "<ParkBrakeApplyCmd>"

== system ElectricalSystem_Test/Subsystem/Testing/BD_ElectricalSystem_Out_Vehicle_SignalSys/ExtractData ==
  In1 : Inport  Partition=on  PartitionDimension=1  PartitionWidth=1  PartitionOffset=0
  Bus Selector : BusSelector  OutputSignals=ATCPower,TrainIntegrity,CabActive,ForwardCoast,BrakeApplied,TractionSafe,EBNotApplied,ModeUpRequest,ModeDownRequest,ModeConfirmRequest,AutomaticChangeEndsRequest,ATOStartRequest,VOBCCutOffSwitch,ASideDoorOpenRequest,BSideDoorOpenRequest,ASideDoorCloseRequest,BSideDoorCloseRequest,AutomaticDoorMode,ManualDoorMode
  For Each : ForEach  DisableCoverage=on
  Out1 : Outport  ConcatenationDimension=1
  Out2 : Outport  Port=2  ConcatenationDimension=1
  Out3 : Outport  Port=3  ConcatenationDimension=1
  Out4 : Outport  Port=4  ConcatenationDimension=1
  Out5 : Outport  Port=5  ConcatenationDimension=1
  Out6 : Outport  Port=6  ConcatenationDimension=1
  Out7 : Outport  Port=7  ConcatenationDimension=1
  Out8 : Outport  Port=8  ConcatenationDimension=1
  Out9 : Outport  Port=9  ConcatenationDimension=1
  Out10 : Outport  Port=10  ConcatenationDimension=1
  Out11 : Outport  Port=11  ConcatenationDimension=1
  Out12 : Outport  Port=12  ConcatenationDimension=1
  Out13 : Outport  Port=13  ConcatenationDimension=1
  Out14 : Outport  Port=14  ConcatenationDimension=1
  Out15 : Outport  Port=15  ConcatenationDimension=1
  Out16 : Outport  Port=16  ConcatenationDimension=1
  Out17 : Outport  Port=17  ConcatenationDimension=1
  Out18 : Outport  Port=18  ConcatenationDimension=1
  Out19 : Outport  Port=19  ConcatenationDimension=1
  wires:
  Bus Selector/8 -> Out8/1  "<ModeUpRequest>"
  Bus Selector/7 -> Out7/1  "<EBNotApplied>"
  Bus Selector/6 -> Out6/1  "<TractionSafe>"
  Bus Selector/5 -> Out5/1  "<BrakeApplied>"
  Bus Selector/4 -> Out4/1  "<ForwardCoast>"
  Bus Selector/3 -> Out3/1  "<CabActive>"
  Bus Selector/2 -> Out2/1  "<TrainIntegrity>"
  Bus Selector/1 -> Out1/1  "<ATCPower>"
  In1/1 -> Bus Selector/1
  Bus Selector/9 -> Out9/1  "<ModeDownRequest>"
  Bus Selector/10 -> Out10/1  "<ModeConfirmRequest>"
  Bus Selector/11 -> Out11/1  "<AutomaticChangeEndsRequest>"
  Bus Selector/12 -> Out12/1  "<ATOStartRequest>"
  Bus Selector/13 -> Out13/1  "<VOBCCutOffSwitch>"
  Bus Selector/14 -> Out14/1  "<ASideDoorOpenRequest>"
  Bus Selector/15 -> Out15/1  "<BSideDoorOpenRequest>"
  Bus Selector/16 -> Out16/1  "<ASideDoorCloseRequest>"
  Bus Selector/17 -> Out17/1  "<BSideDoorCloseRequest>"
  Bus Selector/18 -> Out18/1  "<AutomaticDoorMode>"
  Bus Selector/19 -> Out19/1  "<ManualDoorMode>"

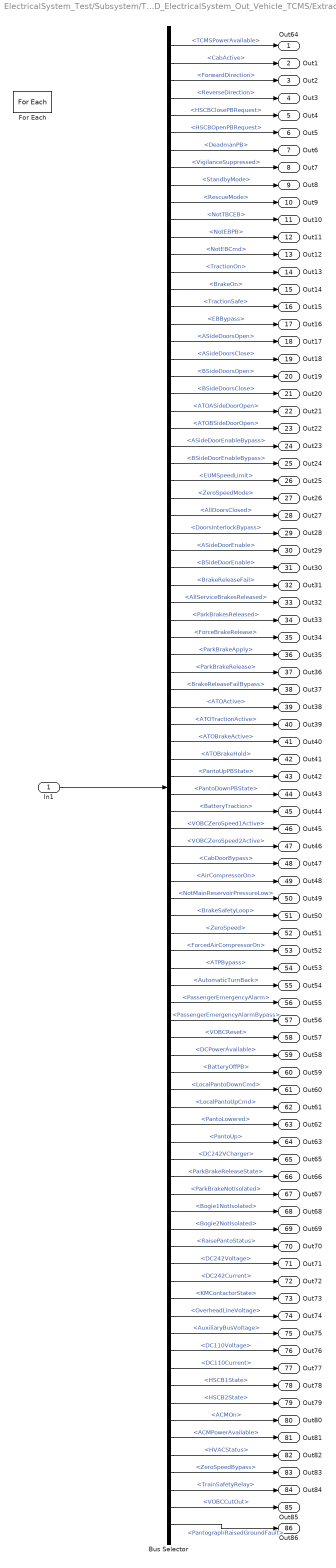
== system ElectricalSystem_Test/Subsystem/Testing/BD_ElectricalSystem_Out_Vehicle_TCMS/ExtractData ==
  In1 : Inport  Partition=on  PartitionDimension=1  PartitionWidth=1  PartitionOffset=0
  Bus Selector : BusSelector  OutputSignals=TCMSPowerAvailable,CabActive,ForwardDirection,ReverseDirection,HSCBClosePBRequest,HSCBOpenPBRequest,DeadmanPB,VigilanceSuppressed,StandbyMode,RescueMode,NotTBCEB,NotEBPB,NotEBCmd,TractionOn,BrakeOn,TractionSafe,EBBypass,ASideDoorsOpen,ASideDoorsClose,BSideDoorsOpen,BSideDoorsClose,ATOASideDoorOpen,ATOBSideDoorOpen,ASideDoorEnableBypass,BSideDoorEnableBypass,EUMSpeedLimit,ZeroSpeedMode,AllDoorsClosed,DoorsInterlockBypass,ASideDoorEnable,BSideDoorEnable,BrakeReleaseFail,AllServiceBrakesReleased,ParkBrakesReleased,ForceBrakeRelease,ParkBrakeApply,ParkBrakeRelease,BrakeReleaseFailBypass,ATOActive,ATOTractionActive,ATOBrakeActive,ATOBrakeHold,PantoUpPBState,PantoDownPBState,BatteryTraction,VOBCZeroSpeed1Active,VOBCZeroSpeed2Active,CabDoorBypass,AirCompressorOn,NotMainReservoirPressureLow,BrakeSafetyLoop,ZeroSpeed,ForcedAirCompressorOn,ATPBypass,AutomaticTurnBack,PassengerEmergencyAlarm,PassengerEmergencyAlarmBypass,VOBCReset,DCPowerAvailable,BatteryOffPB,LocalPantoDownCmd,LocalPantoUpCmd,PantoLowered,PantoUp,DC242VCharger,ParkBrakeReleaseState,ParkBrakeNotIsolated,Bogie1NotIsolated,Bogie2NotIsolated,RaisePantoStatus,DC242Voltage,DC242Current,KMContactorState,OverheadLineVoltage,AuxiliaryBusVoltage,DC110Voltage,DC110Current,HSCB1State,HSCB2State,ACMOn,ACMPowerAvailable,HVACStatus,ZeroSpeedBypass,TrainSafetyRelay,VOBCCutOut,PantographRaisedGroundFault
  For Each : ForEach  DisableCoverage=on
  Out64 : Outport  ConcatenationDimension=1
  Out1 : Outport  Port=2  ConcatenationDimension=1
  Out2 : Outport  Port=3  ConcatenationDimension=1
  Out3 : Outport  Port=4  ConcatenationDimension=1
  Out4 : Outport  Port=5  ConcatenationDimension=1
  Out5 : Outport  Port=6  ConcatenationDimension=1
  Out6 : Outport  Port=7  ConcatenationDimension=1
  Out7 : Outport  Port=8  ConcatenationDimension=1
  Out8 : Outport  Port=9  ConcatenationDimension=1
  Out9 : Outport  Port=10  ConcatenationDimension=1
  Out10 : Outport  Port=11  ConcatenationDimension=1
  Out11 : Outport  Port=12  ConcatenationDimension=1
  Out12 : Outport  Port=13  ConcatenationDimension=1
  Out13 : Outport  Port=14  ConcatenationDimension=1
  Out14 : Outport  Port=15  ConcatenationDimension=1
  Out15 : Outport  Port=16  ConcatenationDimension=1
  Out16 : Outport  Port=17  ConcatenationDimension=1
  Out17 : Outport  Port=18  ConcatenationDimension=1
  Out18 : Outport  Port=19  ConcatenationDimension=1
  Out19 : Outport  Port=20  ConcatenationDimension=1
  Out20 : Outport  Port=21  ConcatenationDimension=1
  Out21 : Outport  Port=22  ConcatenationDimension=1
  Out22 : Outport  Port=23  ConcatenationDimension=1
  Out23 : Outport  Port=24  ConcatenationDimension=1
  Out24 : Outport  Port=25  ConcatenationDimension=1
  Out25 : Outport  Port=26  ConcatenationDimension=1
  Out26 : Outport  Port=27  ConcatenationDimension=1
  Out27 : Outport  Port=28  ConcatenationDimension=1
  Out28 : Outport  Port=29  ConcatenationDimension=1
  Out29 : Outport  Port=30  ConcatenationDimension=1
  Out30 : Outport  Port=31  ConcatenationDimension=1
  Out31 : Outport  Port=32  ConcatenationDimension=1
  Out32 : Outport  Port=33  ConcatenationDimension=1
  Out33 : Outport  Port=34  ConcatenationDimension=1
  Out34 : Outport  Port=35  ConcatenationDimension=1
  Out35 : Outport  Port=36  ConcatenationDimension=1
  Out36 : Outport  Port=37  ConcatenationDimension=1
  Out37 : Outport  Port=38  ConcatenationDimension=1
  Out38 : Outport  Port=39  ConcatenationDimension=1
  Out39 : Outport  Port=40  ConcatenationDimension=1
  Out40 : Outport  Port=41  ConcatenationDimension=1
  Out41 : Outport  Port=42  ConcatenationDimension=1
  Out42 : Outport  Port=43  ConcatenationDimension=1
  Out43 : Outport  Port=44  ConcatenationDimension=1
  Out44 : Outport  Port=45  ConcatenationDimension=1
  Out45 : Outport  Port=46  ConcatenationDimension=1
  Out46 : Outport  Port=47  ConcatenationDimension=1
  Out47 : Outport  Port=48  ConcatenationDimension=1
  Out48 : Outport  Port=49  ConcatenationDimension=1
  Out49 : Outport  Port=50  ConcatenationDimension=1
  Out50 : Outport  Port=51  ConcatenationDimension=1
  Out51 : Outport  Port=52  ConcatenationDimension=1
  Out52 : Outport  Port=53  ConcatenationDimension=1
  Out53 : Outport  Port=54  ConcatenationDimension=1
  Out54 : Outport  Port=55  ConcatenationDimension=1
  Out55 : Outport  Port=56  ConcatenationDimension=1
  Out56 : Outport  Port=57  ConcatenationDimension=1
  Out57 : Outport  Port=58  ConcatenationDimension=1
  Out58 : Outport  Port=59  ConcatenationDimension=1
  Out59 : Outport  Port=60  ConcatenationDimension=1
  Out60 : Outport  Port=61  ConcatenationDimension=1
  Out61 : Outport  Port=62  ConcatenationDimension=1
  Out62 : Outport  Port=63  ConcatenationDimension=1
  Out63 : Outport  Port=64  ConcatenationDimension=1
  Out65 : Outport  Port=65  ConcatenationDimension=1
  Out66 : Outport  Port=66  ConcatenationDimension=1
  Out67 : Outport  Port=67  ConcatenationDimension=1
  Out68 : Outport  Port=68  ConcatenationDimension=1
  Out69 : Outport  Port=69  ConcatenationDimension=1
  Out70 : Outport  Port=70  ConcatenationDimension=1
  Out71 : Outport  Port=71  ConcatenationDimension=1
  Out72 : Outport  Port=72  ConcatenationDimension=1
  Out73 : Outport  Port=73  ConcatenationDimension=1
  Out74 : Outport  Port=74  ConcatenationDimension=1
  Out75 : Outport  Port=75  ConcatenationDimension=1
  Out76 : Outport  Port=76  ConcatenationDimension=1
  Out77 : Outport  Port=77  ConcatenationDimension=1
  Out78 : Outport  Port=78  ConcatenationDimension=1
  Out79 : Outport  Port=79  ConcatenationDimension=1
  Out80 : Outport  Port=80  ConcatenationDimension=1
  Out81 : Outport  Port=81  ConcatenationDimension=1
  Out82 : Outport  Port=82  ConcatenationDimension=1
  Out83 : Outport  Port=83  ConcatenationDimension=1
  Out84 : Outport  Port=84  ConcatenationDimension=1
  Out85 : Outport  Port=85  ConcatenationDimension=1
  Out86 : Outport  Port=86  ConcatenationDimension=1
  wires:
  In1/1 -> Bus Selector/1
  Bus Selector/2 -> Out1/1  "<CabActive>"
  Bus Selector/3 -> Out2/1  "<ForwardDirection>"
  Bus Selector/4 -> Out3/1  "<ReverseDirection>"
  Bus Selector/5 -> Out4/1  "<HSCBClosePBRequest>"
  Bus Selector/6 -> Out5/1  "<HSCBOpenPBRequest>"
  Bus Selector/7 -> Out6/1  "<DeadmanPB>"
  Bus Selector/8 -> Out7/1  "<VigilanceSuppressed>"
  Bus Selector/9 -> Out8/1  "<StandbyMode>"
  Bus Selector/10 -> Out9/1  "<RescueMode>"
  Bus Selector/11 -> Out10/1  "<NotTBCEB>"
  Bus Selector/12 -> Out11/1  "<NotEBPB>"
  Bus Selector/13 -> Out12/1  "<NotEBCmd>"
  Bus Selector/14 -> Out13/1  "<TractionOn>"
  Bus Selector/15 -> Out14/1  "<BrakeOn>"
  Bus Selector/16 -> Out15/1  "<TractionSafe>"
  Bus Selector/17 -> Out16/1  "<EBBypass>"
  Bus Selector/18 -> Out17/1  "<ASideDoorsOpen>"
  Bus Selector/19 -> Out18/1  "<ASideDoorsClose>"
  Bus Selector/20 -> Out19/1  "<BSideDoorsOpen>"
  Bus Selector/21 -> Out20/1  "<BSideDoorsClose>"
  Bus Selector/22 -> Out21/1  "<ATOASideDoorOpen>"
  Bus Selector/23 -> Out22/1  "<ATOBSideDoorOpen>"
  Bus Selector/24 -> Out23/1  "<ASideDoorEnableBypass>"
  Bus Selector/25 -> Out24/1  "<BSideDoorEnableBypass>"
  Bus Selector/26 -> Out25/1  "<EUMSpeedLimit>"
  Bus Selector/27 -> Out26/1  "<ZeroSpeedMode>"
  Bus Selector/28 -> Out27/1  "<AllDoorsClosed>"
  Bus Selector/29 -> Out28/1  "<DoorsInterlockBypass>"
  Bus Selector/30 -> Out29/1  "<ASideDoorEnable>"
  Bus Selector/31 -> Out30/1  "<BSideDoorEnable>"
  Bus Selector/32 -> Out31/1  "<BrakeReleaseFail>"
  Bus Selector/33 -> Out32/1  "<AllServiceBrakesReleased>"
  Bus Selector/34 -> Out33/1  "<ParkBrakesReleased>"
  Bus Selector/35 -> Out34/1  "<ForceBrakeRelease>"
  Bus Selector/36 -> Out35/1  "<ParkBrakeApply>"
  Bus Selector/37 -> Out36/1  "<ParkBrakeRelease>"
  Bus Selector/38 -> Out37/1  "<BrakeReleaseFailBypass>"
  Bus Selector/39 -> Out38/1  "<ATOActive>"
  Bus Selector/40 -> Out39/1  "<ATOTractionActive>"
  Bus Selector/41 -> Out40/1  "<ATOBrakeActive>"
  Bus Selector/42 -> Out41/1  "<ATOBrakeHold>"
  Bus Selector/43 -> Out42/1  "<PantoUpPBState>"
  Bus Selector/44 -> Out43/1  "<PantoDownPBState>"
  Bus Selector/45 -> Out44/1  "<BatteryTraction>"
  Bus Selector/46 -> Out45/1  "<VOBCZeroSpeed1Active>"
  Bus Selector/47 -> Out46/1  "<VOBCZeroSpeed2Active>"
  Bus Selector/48 -> Out47/1  "<CabDoorBypass>"
  Bus Selector/49 -> Out48/1  "<AirCompressorOn>"
  Bus Selector/50 -> Out49/1  "<NotMainReservoirPressureLow>"
  Bus Selector/51 -> Out50/1  "<BrakeSafetyLoop>"
  Bus Selector/52 -> Out51/1  "<ZeroSpeed>"
  Bus Selector/53 -> Out52/1  "<ForcedAirCompressorOn>"
  Bus Selector/54 -> Out53/1  "<ATPBypass>"
  Bus Selector/55 -> Out54/1  "<AutomaticTurnBack>"
  Bus Selector/56 -> Out55/1  "<PassengerEmergencyAlarm>"
  Bus Selector/57 -> Out56/1  "<PassengerEmergencyAlarmBypass>"
  Bus Selector/58 -> Out57/1  "<VOBCReset>"
  Bus Selector/59 -> Out58/1  "<DCPowerAvailable>"
  Bus Selector/60 -> Out59/1  "<BatteryOffPB>"
  Bus Selector/61 -> Out60/1  "<LocalPantoDownCmd>"
  Bus Selector/62 -> Out61/1  "<LocalPantoUpCmd>"
  Bus Selector/63 -> Out62/1  "<PantoLowered>"
  Bus Selector/64 -> Out63/1  "<PantoUp>"
  Bus Selector/65 -> Out65/1  "<DC242VCharger>"
  Bus Selector/66 -> Out66/1  "<ParkBrakeReleaseState>"
  Bus Selector/67 -> Out67/1  "<ParkBrakeNotIsolated>"
  Bus Selector/68 -> Out68/1  "<Bogie1NotIsolated>"
  Bus Selector/69 -> Out69/1  "<Bogie2NotIsolated>"
  Bus Selector/70 -> Out70/1  "<RaisePantoStatus>"
  Bus Selector/71 -> Out71/1  "<DC242Voltage>"
  Bus Selector/72 -> Out72/1  "<DC242Current>"
  Bus Selector/73 -> Out73/1  "<KMContactorState>"
  Bus Selector/74 -> Out74/1  "<OverheadLineVoltage>"
  Bus Selector/75 -> Out75/1  "<AuxiliaryBusVoltage>"
  Bus Selector/76 -> Out76/1  "<DC110Voltage>"
  Bus Selector/77 -> Out77/1  "<DC110Current>"
  Bus Selector/78 -> Out78/1  "<HSCB1State>"
  Bus Selector/79 -> Out79/1  "<HSCB2State>"
  Bus Selector/80 -> Out80/1  "<ACMOn>"
  Bus Selector/81 -> Out81/1  "<ACMPowerAvailable>"
  Bus Selector/84 -> Out84/1  "<TrainSafetyRelay>"
  Bus Selector/83 -> Out83/1  "<ZeroSpeedBypass>"
  Bus Selector/82 -> Out82/1  "<HVACStatus>"
  Bus Selector/85 -> Out85/1  "<VOBCCutOut>"
  Bus Selector/1 -> Out64/1  "<TCMSPowerAvailable>"
  Bus Selector/86 -> Out86/1  "<PantographRaisedGroundFault>"

== system ElectricalSystem_Test/Subsystem/Testing/BD_ElectricalSystem_Out_Vehicle_Traction/ExtractData ==
  In1 : Inport  Partition=on  PartitionDimension=1  PartitionWidth=1  PartitionOffset=0
  Bus Selector : BusSelector  OutputSignals=MCMPowerAvailable,MotorPower,HSCBClosePBRequest,HSCBOpenPBRequest,ForwardDirection,ReverseDirection,ReverseSpeedLimit,TBCTraction,TBCNotHighTraction,TBCNotBraking,TractionSafe,ForceBrakeRelease,BackupModeCmd,AllBrakesReleased,BatteryTractionRequest,EmergencyInverterWorking
  For Each : ForEach  DisableCoverage=on
  Out : Outport  ConcatenationDimension=1
  Out1 : Outport  Port=2  ConcatenationDimension=1
  Out2 : Outport  Port=3  ConcatenationDimension=1
  Out3 : Outport  Port=4  ConcatenationDimension=1
  Out4 : Outport  Port=5  ConcatenationDimension=1
  Out5 : Outport  Port=6  ConcatenationDimension=1
  Out6 : Outport  Port=7  ConcatenationDimension=1
  Out7 : Outport  Port=8  ConcatenationDimension=1
  Out8 : Outport  Port=9  ConcatenationDimension=1
  Out9 : Outport  Port=10  ConcatenationDimension=1
  Out10 : Outport  Port=11  ConcatenationDimension=1
  Out11 : Outport  Port=12  ConcatenationDimension=1
  Out12 : Outport  Port=13  ConcatenationDimension=1
  Out13 : Outport  Port=14  ConcatenationDimension=1
  Out14 : Outport  Port=15  ConcatenationDimension=1
  Out15 : Outport  Port=16  ConcatenationDimension=1
  wires:
  In1/1 -> Bus Selector/1
  Bus Selector/1 -> Out/1  "<MCMPowerAvailable>"
  Bus Selector/2 -> Out1/1  "<MotorPower>"
  Bus Selector/3 -> Out2/1  "<HSCBClosePBRequest>"
  Bus Selector/4 -> Out3/1  "<HSCBOpenPBRequest>"
  Bus Selector/5 -> Out4/1  "<ForwardDirection>"
  Bus Selector/6 -> Out5/1  "<ReverseDirection>"
  Bus Selector/7 -> Out6/1  "<ReverseSpeedLimit>"
  Bus Selector/8 -> Out7/1  "<TBCTraction>"
  Bus Selector/9 -> Out8/1  "<TBCNotHighTraction>"
  Bus Selector/10 -> Out9/1  "<TBCNotBraking>"
  Bus Selector/11 -> Out10/1  "<TractionSafe>"
  Bus Selector/12 -> Out11/1  "<ForceBrakeRelease>"
  Bus Selector/13 -> Out12/1  "<BackupModeCmd>"
  Bus Selector/14 -> Out13/1  "<AllBrakesReleased>"
  Bus Selector/16 -> Out15/1  "<EmergencyInverterWorking>"
  Bus Selector/15 -> Out14/1  "<BatteryTractionRequest>"

== system ElectricalSystem_Test/Subsystem/Testing/Subsystem/For Each Subsystem ==
  In1 : Inport  Partition=on  PartitionDimension=1  PartitionWidth=1  PartitionOffset=0
  Bus Selector : BusSelector  OutputSignals=OutputControlStates,Traction,Braking,TCMS,Pneumatics,SignalSys,Doors,Audio
  For Each : ForEach  DisableCoverage=on
  Out1 : Outport  ConcatenationDimension=1
  Out2 : Outport  Port=2  ConcatenationDimension=1
  Out3 : Outport  Port=3  ConcatenationDimension=1
  Out5 : Outport  Port=4  ConcatenationDimension=1
  Out6 : Outport  Port=5  ConcatenationDimension=1
  Out7 : Outport  Port=6  ConcatenationDimension=1
  Out8 : Outport  Port=7  ConcatenationDimension=1
  Out4 : Outport  Port=8  ConcatenationDimension=1
  wires:
  In1/1 -> Bus Selector/1
  Bus Selector/1 -> Out1/1  "<OutputControlStates>"
  Bus Selector/2 -> Out2/1  "<Traction>"
  Bus Selector/3 -> Out3/1  "<Braking>"
  Bus Selector/4 -> Out5/1  "<TCMS>"
  Bus Selector/5 -> Out6/1  "<Pneumatics>"
  Bus Selector/6 -> Out7/1  "<SignalSys>"
  Bus Selector/7 -> Out8/1  "<Doors>"
  Bus Selector/8 -> Out4/1  "<Audio>"
